simulink model "Global_Nocontrol"  (R2016a)
settings: Solver=ode8  StartTime=0.0  StopTime=1400  FixedStep=1  RelTol=1e-3
(part 2 of 2)

== matlab function Global_Nocontrol/Subsystem2/Height and Volume ==
  data: Qin input; A input; dH output; Qout input
function dH  = Height_and_Volume(Qin,A,Qout)
    dH = (Qin-Qout)*(1/A);
end

== matlab function Global_Nocontrol/Subsystem2/Overflow  ==
  data: H input; Q_overflow output; Qin input; Overflow_Height input
function Q_overflow = fcn(H,Qin,Overflow_Height)
%#codegen
if H>=Overflow_Height;
    Q_overflow=Qin;
else 
    Q_overflow=0;
end

== matlab function Global_Nocontrol/Subsystem2/Oxygen Control/ Oxygen Setpoint1 ==
  data: Height input; Intergration_Control output; Integration_Control1 output; Integration_Control2 output
function [Intergration_Control,Integration_Control1,Integration_Control2] = fcn(Height)
if Height>0 
    Intergration_Control=0;
else 
    Intergration_Control=1;
end
    
if Height>0.25
    Integration_Control1=0;
else 
    Integration_Control1=1;
end
if Height>0.75
    Integration_Control2=0;
else 
    Integration_Control2=1;
end

== matlab function Global_Nocontrol/Subsystem2/Oxygen Control/0 to 0.25/ Nitrate ==
  data: Oxygen_Level input; K_Nitrate output; K_Nitr input
function K_Nitrate = fcn(Oxygen_Level,K_Nitr)

if Oxygen_Level< 1.0
    K_Nitrate = K_Nitr;
else
    K_Nitrate = 0;
end

== matlab function Global_Nocontrol/Subsystem2/Oxygen Control/0 to 0.25/ Oxygen Control ==
  data: c input; dOxygen_Level output; K input
function dOxygen_Level = fcn(c,K)

dOxygen_Level = -c * K;

== matlab function Global_Nocontrol/Subsystem2/Q out ==
  data: H input; Qout output; Control_Height input
function Qout = fcn(H,Control_Height)

if H<=Control_Height
    Qout=0;
else
    
   Qout = sqrt(2*9.81*H);
   

end

== matlab function Global_Nocontrol/Wetland/Oxygen Control/0.25 ro 0.75/ Nitrate ==
  data: Oxygen_Level input; K_Nitrate output; K_Nitr input
function K_Nitrate = fcn(Oxygen_Level,K_Nitr)

if Oxygen_Level< 1.0
    K_Nitrate = K_Nitr;
else
    K_Nitrate = 0;
end

== matlab function Global_Nocontrol/Wetland/Oxygen Control/0.25 ro 0.75/ Oxygen Control ==
  data: c input; dOxygen_Level output; K input
function dOxygen_Level = fcn(c,K)

dOxygen_Level = -c * K;

== matlab function Global_Nocontrol/Wetland/Oxygen Control/0.75 / Nitrate ==
  data: Oxygen_Level input; K_Nitrate output; K_Nitr input
function K_Nitrate = fcn(Oxygen_Level,K_Nitr)

if Oxygen_Level< 1.0
    K_Nitrate = K_Nitr;
else
    K_Nitrate = 0;
end

== matlab function Global_Nocontrol/Subsystem3/Oxygen Control/0.25 ro 0.75/ Nitrate ==
  data: Oxygen_Level input; K_Nitrate output; K_Nitr input
function K_Nitrate = fcn(Oxygen_Level,K_Nitr)

if Oxygen_Level< 1.0
    K_Nitrate = K_Nitr;
else
    K_Nitrate = 0;
end

== matlab function Global_Nocontrol/Subsystem3/Oxygen Control/0.25 ro 0.75/ Oxygen Control ==
  data: c input; dOxygen_Level output; K input
function dOxygen_Level = fcn(c,K)

dOxygen_Level = -c * K;

== matlab function Global_Nocontrol/Subsystem3/Oxygen Control/0.75 / Nitrate ==
  data: Oxygen_Level input; K_Nitrate output; K_Nitr input
function K_Nitrate = fcn(Oxygen_Level,K_Nitr)

if Oxygen_Level< 1.0
    K_Nitrate = K_Nitr;
else
    K_Nitrate = 0;
end

== matlab function Global_Nocontrol/Subsystem3/Oxygen Control/0.75 / Oxygen Control ==
  data: c input; dOxygen_Level output; K input
function dOxygen_Level = fcn(c,K)

dOxygen_Level = -c * K;

== matlab function Global_Nocontrol/Subsystem2/Oxygen Control/0.25 ro 0.75/ Nitrate ==
  data: Oxygen_Level input; K_Nitrate output; K_Nitr input
function K_Nitrate = fcn(Oxygen_Level,K_Nitr)

if Oxygen_Level< 1.0
    K_Nitrate = K_Nitr;
else
    K_Nitrate = 0;
end

== matlab function Global_Nocontrol/Subsystem2/Oxygen Control/0.25 ro 0.75/ Oxygen Control ==
  data: c input; dOxygen_Level output; K input
function dOxygen_Level = fcn(c,K)

dOxygen_Level = -c * K;

== matlab function Global_Nocontrol/Subsystem2/Oxygen Control/0.75 / Nitrate ==
  data: Oxygen_Level input; K_Nitrate output; K_Nitr input
function K_Nitrate = fcn(Oxygen_Level,K_Nitr)

if Oxygen_Level< 1.0
    K_Nitrate = K_Nitr;
else
    K_Nitrate = 0;
end

== matlab function Global_Nocontrol/Subsystem2/Oxygen Control/0.75 / Oxygen Control ==
  data: c input; dOxygen_Level output; K input
function dOxygen_Level = fcn(c,K)

dOxygen_Level = -c * K;

== matlab function Global_Nocontrol/Subsystem1/Oxygen Control/0.25 ro 0.75/ Nitrate ==
  data: Oxygen_Level input; K_Nitrate output; K_Nitr input
function K_Nitrate = fcn(Oxygen_Level,K_Nitr)

if Oxygen_Level< 1.0
    K_Nitrate = K_Nitr;
else
    K_Nitrate = 0;
end

== matlab function Global_Nocontrol/Subsystem1/Oxygen Control/0.25 ro 0.75/ Oxygen Control ==
  data: c input; dOxygen_Level output; K input
function dOxygen_Level = fcn(c,K)

dOxygen_Level = -c * K;

== matlab function Global_Nocontrol/Subsystem1/Oxygen Control/0.75 / Nitrate ==
  data: Oxygen_Level input; K_Nitrate output; K_Nitr input
function K_Nitrate = fcn(Oxygen_Level,K_Nitr)

if Oxygen_Level< 1.0
    K_Nitrate = K_Nitr;
else
    K_Nitrate = 0;
end

== matlab function Global_Nocontrol/Subsystem1/Oxygen Control/0.75 / Oxygen Control ==
  data: c input; dOxygen_Level output; K input
function dOxygen_Level = fcn(c,K)

dOxygen_Level = -c * K;

== matlab function Global_Nocontrol/Wetland/Oxygen Control/0.75 / Oxygen Control ==
  data: c input; dOxygen_Level output; K input
function dOxygen_Level = fcn(c,K)

dOxygen_Level = -c * K;

== matlab function Global_Nocontrol/Wetland/Oxygen Control/ 1.5/ Nitrate ==
  data: Oxygen_Level input; K_Nitrate output; K_Nitr input
function K_Nitrate = fcn(Oxygen_Level,K_Nitr)

if Oxygen_Level< 1.0
    K_Nitrate = K_Nitr;
else
    K_Nitrate = 0;
end

== matlab function Global_Nocontrol/Wetland/Oxygen Control/ 1.5/ Oxygen Control ==
  data: c input; dOxygen_Level output; K input
function dOxygen_Level = fcn(c,K)

dOxygen_Level = -c * K;
